simulink model "gazeboExampleStateflow"  (R2017b)
settings: Solver=FixedStepDiscrete  StartTime=0.0  StopTime=inf  FixedStep=params.Ts  RelTol=1e-3  EnableMultiTasking=on
PreLoadFcn:
  | params = controlParamsGazebo;
  | 
  | rosshutdown;
  | loadIpAddresses;
  | rosinit(gazeboIp);
model workspace (MAT data in the model file):
  SL_ROS_VariableLengthArrays_MaxSizes.CommonInfo.ArrayTruncateAction = 'EmitWarning'
  SL_ROS_VariableLengthArrays_MaxSizes.MsgTypeMap = containers.Map
  SL_ROS_VariableLengthArrays_MaxSizes.MsgTypeMap.serialization.keys = {'sensor_msgs/Image'}
  SL_ROS_VariableLengthArrays_MaxSizes.MsgTypeMap.serialization.values{1}(1).PropertyName = 'Data'
  SL_ROS_VariableLengthArrays_MaxSizes.MsgTypeMap.serialization.values{1}(1).DataType = 'uint8'
  SL_ROS_VariableLengthArrays_MaxSizes.MsgTypeMap.serialization.values{1}(1).MaxLength = 921600
  SL_ROS_VariableLengthArrays_MaxSizes.MsgTypeMap.serialization.values{1}(2).PropertyName = 'Encoding'
  SL_ROS_VariableLengthArrays_MaxSizes.MsgTypeMap.serialization.values{1}(2).DataType = 'uint8'
  SL_ROS_VariableLengthArrays_MaxSizes.MsgTypeMap.serialization.values{1}(2).MaxLength = 128
  SL_ROS_VariableLengthArrays_MaxSizes.MsgTypeMap.serialization.uniformity = 0
  SL_ROS_VariableLengthArrays_MaxSizes.MsgTypeMap.serialization.keyType = 'char'
  SL_ROS_VariableLengthArrays_MaxSizes.MsgTypeMap.serialization.valueType = 'any'
undefined symbols (not defined in the file): Angular, Linear
libraries: robotlib x4, simulink x2, visiontextngfix x1, visionsinks x1
settings Model: Creator=scastro  LastModifiedBy=scastro
settings SolverCC: PositivePriorityOrder=on
settings OptimizationCC: PassReuseOutputArgsAs=Individual arguments  MaxStackSize=64
settings DebuggingCC: ParameterTunabilityLossMsg=error
settings HardwareCC: ProdBitPerLong=64  ProdHWDeviceType=Intel->x86-64 (Linux 64)
settings RTWCC: SystemTargetFile=ert.tlc  HardwareBoard=Robot Operating System (ROS)  TemplateMakefile=ert_default_tmf  GenerateReport=on  Toolchain=Catkin  IncludeHyperlinkInReport=on  LaunchReport=on  TargetLang=C++  GenerateTraceInfo=on  GenerateTraceReport=on  GenerateTraceReportSl=on  GenerateTraceReportSf=on  GenerateTraceReportEml=on
settings CodeAppCC: ForceParamTrailComments=on  IgnoreCustomStorageClasses=off  OperatorAnnotations=on  SimulinkDataObjDesc=on  SFDataObjDesc=on  MATLABFcnDesc=on  InsertBlockDesc=on  StateflowObjectComments=on  MATLABSourceComments=on
settings ERTTargetCC: SupportVariableSizeSignals=on

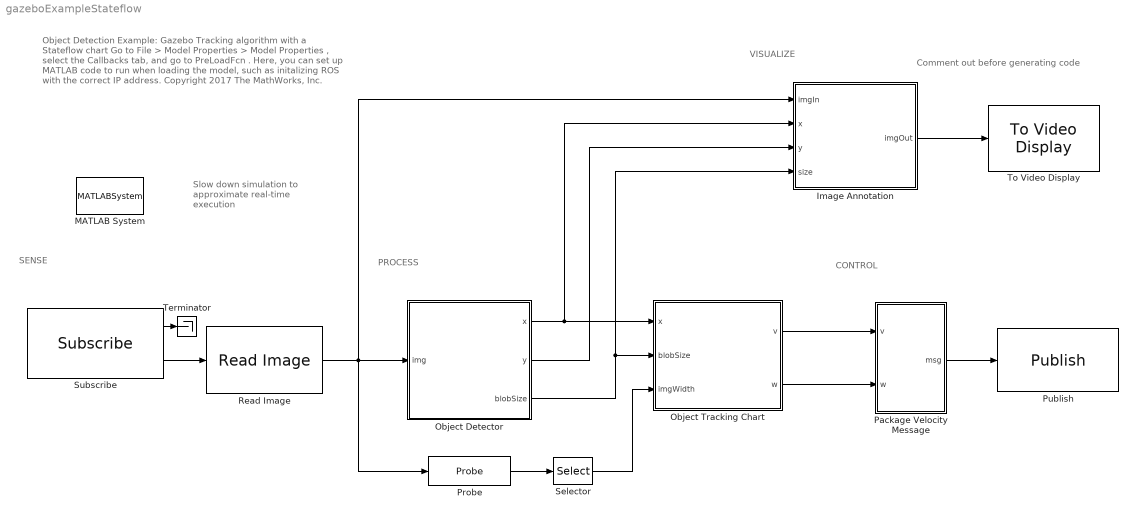
== system gazeboExampleStateflow ==
  note: Comment out before generating code
  note: CONTROL
  note: PROCESS
  note: SENSE
  note: VISUALIZE
  note: Slow down simulation to approximate real-time execution
  note: Object Detection Example: Gazebo
      | Tracking algorithm with a Stateflow chart
      |
      | Go to File > Model Properties > Model Properties , select the Callbacks tab, and go to PreLoadFcn . Here, you can set up MATLAB code to run when loading the model, such as initalizing ROS with the correct IP address.
      |
      | Copyright 2017 The MathWorks, Inc.
  Image Annotation : Subsystem
  MATLAB System : MATLABSystem  System=ExampleHelperSimulationRateControl  SampleTime=params.Ts
      mask Type: ExampleHelperSimulationRateControl
      mask Display: disp('Rate Control');
  Object Detector : MATLAB Function  TreatAsAtomicUnit=on
  Object Tracking Chart : Stateflow chart  TreatAsAtomicUnit=on
  Package Velocity Message : Subsystem
  Probe : Probe  ProbeWidth=off  ProbeSampleTime=off  ProbeComplexSignal=off  ProbeSignalDimensions=on
  Publish : robotlib/Publish  SourceLibraryInfo=This block requires Robotics System Toolbox  topicSource=Select from ROS network  topic=/mobile_base/commands/velocity  messageType=geometry_msgs/Twist  messageQueueLength=1
      settings: SourceProductBaseCode=RO
  Read Image : robotlib/Read Image  SourceLibraryInfo=This block requires Robotics System Toolbox  MaximumImageSize=[480, 640]  ImageEncoding=rgb8  ShowAlphaOutput=off  ShowErrorCodeOutput=off  VariableSizeOutputs=off
      settings: SourceProductName=Robotics System Toolbox  SourceProductBaseCode=RO
  Selector : Selector  InputPortWidth=3  IndexOptions=Index vector (dialog)  Indices=2  OutputSizes=1
  Subscribe : robotlib/Subscribe  SourceLibraryInfo=This block requires Robotics System Toolbox  topicSource=Select from ROS network  topic=/camera/rgb/image_raw  messageType=sensor_msgs/Image  sampleTime=-1  messageQueueLength=1
      settings: SourceProductBaseCode=RO
  Terminator : Terminator
  To Video Display : visionsinks/To Video Display  windowSizeMode=Normal  openAtMdlStart=on  fullScreen=off  videoWindowX=665  videoWindowY=103  saveWindowSize=off  videoWindowWidth=691  videoWindowHeight=561  inputColorFormat=RGB  inputType=Obsolete  imagePorts=One multidimensional signal  OutputDevice=On-screen video monitor  dataOrg=Column-major  isWindowOpen=off
      settings: SourceProductName=Computer Vision System Toolbox
  wires:
  Object Detector/3(blobSize) -> Object Tracking Chart/2(blobSize), Image Annotation/4(size)
  Object Detector/1(x) -> Object Tracking Chart/1(x), Image Annotation/2(x)
  Image Annotation/1(imgOut) -> To Video Display/1
  Probe/1 -> Selector/1
  Selector/1 -> Object Tracking Chart/3(imgWidth)
  Object Tracking Chart/1(v) -> Package Velocity Message/1(v)
  Object Tracking Chart/2(w) -> Package Velocity Message/2(w)
  Package Velocity Message/1(msg) -> Publish/1
  Subscribe/2 -> Read Image/1
  Object Detector/2(y) -> Image Annotation/3(y)
  Read Image/1 -> Object Detector/1(img), Image Annotation/1(imgIn), Probe/1
  Subscribe/1 -> Terminator/1

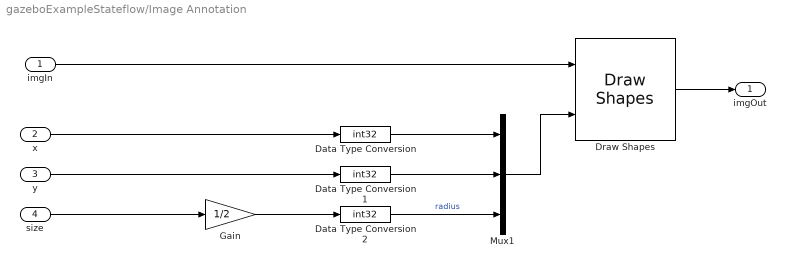
== system gazeboExampleStateflow/Image Annotation ==
  imgIn : Inport
  x : Inport  Port=2
  y : Inport  Port=3
  size : Inport  Port=4
  Data Type Conversion : DataTypeConversion  OutDataTypeStr=int32
  Data Type Conversion1 : DataTypeConversion  OutDataTypeStr=int32
  Data Type Conversion2 : DataTypeConversion  OutDataTypeStr=int32
  Draw Shapes : visiontextngfix/Draw Shapes  shape=Circles  fill=off  lineWidth=2  fillClrSource=Specify via dialog  display=User-specified value  intensity=200  color=[255 255 0]  opacity=0.6  viewport=Entire image  antialiasing=off  inType=Obsolete  imagePorts=One multidimensional signal  prodOutputMode=Binary point scaling  prodOutputWordLength=32  prodOutputFracLength=14  memoryMode=Specify word length  memoryWordLength=16  memoryFracLength=14  roundingMode=Floor  overflowMode=off
      settings: SourceProductName=Computer Vision System Toolbox
  Gain : Gain  Gain=1/2
  Mux1 : Mux  Inputs=3
  imgOut : Outport
  wires:
  y/1 -> Data Type Conversion1/1
  Data Type Conversion1/1 -> Mux1/2
  Data Type Conversion/1 -> Mux1/1
  x/1 -> Data Type Conversion/1
  imgIn/1 -> Draw Shapes/1
  Draw Shapes/1 -> imgOut/1
  Mux1/1 -> Draw Shapes/2
  Gain/1 -> Data Type Conversion2/1
  size/1 -> Gain/1
  Data Type Conversion2/1 -> Mux1/3  "radius"

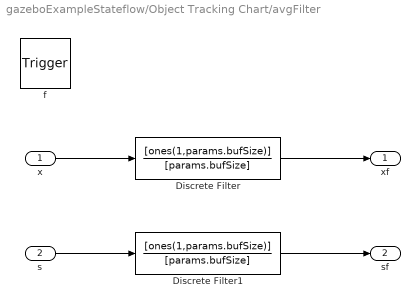
== system gazeboExampleStateflow/Object Tracking Chart/avgFilter ==
  x : Inport  OutDataTypeStr=double  PortDimensions=1
  s : Inport  Port=2  OutDataTypeStr=double  PortDimensions=1
  f : TriggerPort  TriggerType=function-call  VariantControl=Variant
      settings: CopyFcn=Stateflow.SLINSF.SimulinkMan.removeBlockPreDeleteFcn  PreDeleteFcn=Stateflow.SLINSF.SimulinkMan.unsafePredeleteFcn
  Discrete Filter : DiscreteFilter  Numerator=[ones(1,params.bufSize)]  Denominator=[params.bufSize]
  Discrete Filter1 : DiscreteFilter  Numerator=[ones(1,params.bufSize)]  Denominator=[params.bufSize]
  xf : Outport
  sf : Outport  Port=2
  wires:
  x/1 -> Discrete Filter/1
  Discrete Filter/1 -> xf/1
  s/1 -> Discrete Filter1/1
  Discrete Filter1/1 -> sf/1

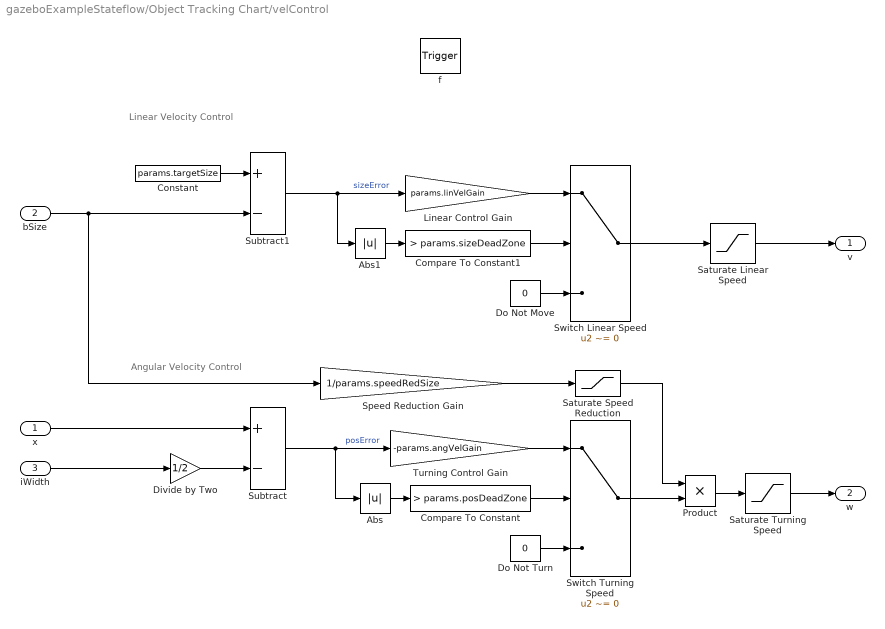
== system gazeboExampleStateflow/Object Tracking Chart/velControl ==
  note: Angular Velocity Control
  note: Linear Velocity Control
  x : Inport  OutDataTypeStr=double  PortDimensions=1
  bSize : Inport  Port=2  OutDataTypeStr=double  PortDimensions=1
  iWidth : Inport  Port=3  OutDataTypeStr=double  PortDimensions=1
  f : TriggerPort  TriggerType=function-call  VariantControl=Variant
      settings: CopyFcn=Stateflow.SLINSF.SimulinkMan.removeBlockPreDeleteFcn  PreDeleteFcn=Stateflow.SLINSF.SimulinkMan.unsafePredeleteFcn
  Abs : Abs
  Abs1 : Abs
  Compare To Constant : simulink/Logic and Bit Operations/Compare To Constant  relop=>  const=params.posDeadZone  OutDataTypeStr=boolean
  Compare To Constant1 : simulink/Logic and Bit Operations/Compare To Constant  relop=>  const=params.sizeDeadZone  OutDataTypeStr=boolean
  Constant : Constant  Value=params.targetSize
  Divide by Two : Gain  Gain=1/2
  Do Not Move : Constant  Value=0
  Do Not Turn : Constant  Value=0
  Linear Control Gain : Gain  Gain=params.linVelGain
  Product : Product
  Saturate Linear Speed : Saturate  UpperLimit=params.maxLinVel  LowerLimit=-params.maxLinVel
  Saturate Speed Reduction : Saturate  UpperLimit=1  LowerLimit=0
  Saturate Turning Speed : Saturate  UpperLimit=params.maxAngVel  LowerLimit=-params.maxAngVel
  Speed Reduction Gain : Gain  Gain=1/params.speedRedSize
  Subtract : Sum  Inputs=+-
  Subtract1 : Sum  Inputs=+-
  Switch Linear Speed : Switch  Criteria=u2 ~= 0
  Switch Turning Speed : Switch  Criteria=u2 ~= 0
  Turning Control Gain : Gain  Gain=-params.angVelGain
  v : Outport  OutputWhenDisabled=reset  InitialOutput=0
  w : Outport  Port=2  OutputWhenDisabled=reset  InitialOutput=0
  wires:
  Compare To Constant/1 -> Switch Turning Speed/2
  Saturate Turning Speed/1 -> w/1
  Saturate Speed Reduction/1 -> Product/1
  Linear Control Gain/1 -> Switch Linear Speed/1
  Do Not Turn/1 -> Switch Turning Speed/3
  Speed Reduction Gain/1 -> Saturate Speed Reduction/1
  bSize/1 -> Subtract1/2, Speed Reduction Gain/1
  Compare To Constant1/1 -> Switch Linear Speed/2
  Saturate Linear Speed/1 -> v/1
  Switch Turning Speed/1 -> Product/2
  Switch Linear Speed/1 -> Saturate Linear Speed/1
  iWidth/1 -> Divide by Two/1
  Abs1/1 -> Compare To Constant1/1
  Turning Control Gain/1 -> Switch Turning Speed/1
  Constant/1 -> Subtract1/1
  Do Not Move/1 -> Switch Linear Speed/3
  Subtract1/1 -> Linear Control Gain/1, Abs1/1  "sizeError"
  Divide by Two/1 -> Subtract/2
  Subtract/1 -> Turning Control Gain/1, Abs/1  "posError"
  Abs/1 -> Compare To Constant/1
  x/1 -> Subtract/1
  Product/1 -> Saturate Turning Speed/1

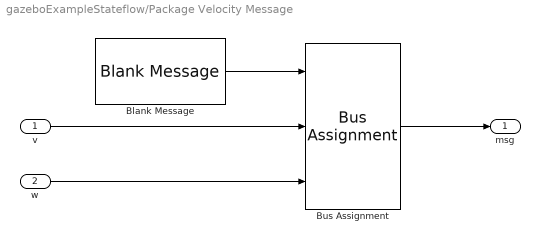
== system gazeboExampleStateflow/Package Velocity Message ==
  v : Inport
  w : Inport  Port=2
  Blank Message : robotlib/Blank Message  SourceLibraryInfo=This block requires Robotics System Toolbox  messageType=geometry_msgs/Twist  SampleTime=inf
      settings: SourceProductBaseCode=RO
  Bus Assignment : BusAssignment  AssignedSignals=Linear.X,Angular.Z
  msg : Outport
  wires:
  Blank Message/1 -> Bus Assignment/1
  Bus Assignment/1 -> msg/1
  w/1 -> Bus Assignment/3
  v/1 -> Bus Assignment/2

== matlab function gazeboExampleStateflow/Object Detector ==
  data: x output; img input; y output; blobSize output
function [x,y,blobSize] = CircleDetection(img)
    
    % Initialize outputs
    x = 0;
    y = 0;
    blobSize = 0;
    
    % Call external function
    resizeScale = 0.5;
    [x,y,blobSize] = detectCircle(img,resizeScale);

end

== stateflow chart gazeboExampleStateflow/Object Tracking Chart ==
  state TrackMarker [parallel]
    en,du:
    [xFilt,sizeFilt] = avgFilter(x,blobSize);
    settings: executionOrder=2
    state Normal
      en,du:
      [v,w] = velControl(xFilt,sizeFilt,imgWidth);
    state Abnormal
      state Scan
        en:
        v = 0;
        w = params.maxAngVel/2;
      state Stop
        en:
        v = 0;
        w = 0;
      (default) -> Scan
      Stop -> Scan : [count >= 50 && ...
          | count <= 500]
      Scan -> Stop : [count >= 500]
    (default) -> Normal
    Normal -> Abnormal : [count >= ...
        | params.maxCounts]
    Abnormal -> Normal : [count < ...
        | params.maxCounts]
  state DetectOutliers [parallel]
    settings: executionOrder=1
    (default) -> (junction 15) : {
        | count = 0;
        | xPrev = 0;
        | }
    DetectOutliers -> (junction 15)
    (junction 15) -> (junction 16) [order 1] : % Test for outlier
        | [abs(x-xPrev)>=params.maxDisp || ...
        | blobSize<=params.minSize || ...
        | blobSize>=params.maxSize]
    (junction 15) -> (junction 19) [order 2] : % Reset counter
        | {count = 0;}
    (junction 16) -> (junction 24) : % Increment counter
        | % with saturation
    (junction 24) -> (junction 27) [order 1] : [count<1000]
    (junction 24) -> (junction 21) [order 2]
    (junction 27) -> (junction 29) : {count=count+1;}
    (junction 21) -> (junction 19)
    (junction 29) -> (junction 21)
    (junction 19) -> (junction 54) : % Update previous location value
        | {xPrev = x;}
  state [xf,sf] = avgFilter(x,s) [function]
  state [v,w] = velControl(x,bSize,iWidth) [function]
  data: x function_input double size=1; s function_input double size=1; xf function_output; sf function_output; x function_input double size=1; bSize function_input double size=1; iWidth function_input double size=1; v function_output; w function_output; x input; blobSize input; imgWidth input; v output; w output; sizeFilt local; xFilt local; count local; xPrev local; params parameter
